simulink model "ModID_R2018a"  (R2018a)
settings: Solver=VariableStepAuto  StartTime=0.0  StopTime=10.0  RelTol=1e-3
values from neighbouring files (symbols this model uses):
  matrcomp =     [theta_sim_nonlinv2.mat]
libraries: dspinverses x1
settings Model: Creator=jannekeblok  LastModifiedBy=jessi
settings DebuggingCC: LibraryContextMissingDiagnostic=warning
settings CodeAppCC: StateflowObjectComments=on

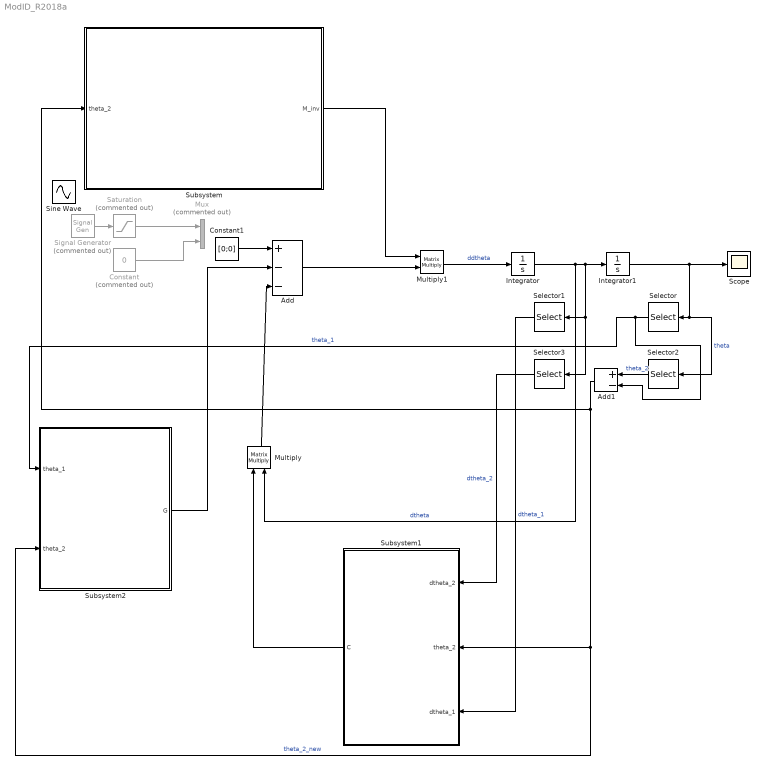
== system ModID_R2018a ==
  Add : Sum  Inputs=+--
  Add1 : Sum  Inputs=+-
  Constant : Constant  Commented=on  Value=0
  Constant1 : Constant  Value=[0;0]
  Integrator : Integrator
  Integrator1 : Integrator  InitialCondition=[pi;3/2*pi]
  Multiply : Product  Multiplication=Matrix(*)
  Multiply1 : Product  Multiplication=Matrix(*)
  Mux : Mux  Commented=on  Inputs=2
  Saturation : Saturate  Commented=on  UpperLimit=1  LowerLimit=-1
  Scope : Scope
  Selector : Selector  InputPortWidth=2  IndexOptions=Index vector (dialog)  Indices=[1]  OutputSizes=1
  Selector1 : Selector  InputPortWidth=2  IndexOptions=Index vector (dialog)  Indices=[1]  OutputSizes=1
  Selector2 : Selector  InputPortWidth=2  IndexOptions=Index vector (dialog)  Indices=[2]  OutputSizes=1
  Selector3 : Selector  InputPortWidth=2  IndexOptions=Index vector (dialog)  Indices=[2]  OutputSizes=1
  Signal Generator : SignalGenerator  Commented=on  Amplitude=0.3*1  Units=rad/sec
  Sine Wave : Sin  SampleTime=0
  Subsystem : Subsystem
  Subsystem1 : Subsystem
  Subsystem2 : Subsystem
  wires:
  Multiply/1 -> Add/3
  Subsystem/1(M_inv) -> Multiply1/1
  Add/1 -> Multiply1/2
  Subsystem1/1(C) -> Multiply/1
  Integrator/1 -> Multiply/2, Selector1/1, Selector3/1, Integrator1/1  "dtheta"
  Selector/1 -> Add1/2, Subsystem2/1(theta_1)  "theta_1"
  Multiply1/1 -> Integrator/1  "ddtheta"
  Constant/1 -> Mux/2
  Selector1/1 -> Subsystem1/3(dtheta_1)  "dtheta_1"
  Constant1/1 -> Add/1
  Selector2/1 -> Add1/1  "theta_2"
  Selector3/1 -> Subsystem1/1(dtheta_2)  "dtheta_2"
  Signal Generator/1 -> Saturation/1
  Integrator1/1 -> Scope/1, Selector2/1, Selector/1  "theta"
  Subsystem2/1(G) -> Add/2
  Saturation/1 -> Mux/1
  Add1/1 -> Subsystem2/2("theta_2 "), Subsystem1/2(theta_2), Subsystem/1("theta_2 ")  "theta_2_new"

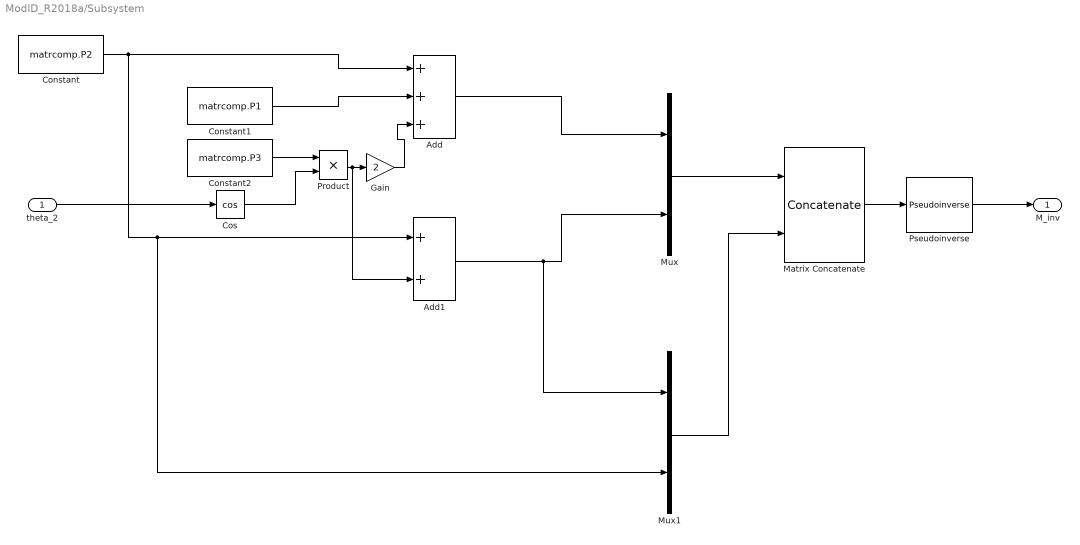
== system ModID_R2018a/Subsystem ==
  "theta_2 " : Inport
  Add : Sum  Inputs=+++
  Add1 : Sum
  Constant : Constant  Value=matrcomp.P2
  Constant1 : Constant  Value=matrcomp.P1
  Constant2 : Constant  Value=matrcomp.P3
  Cos : Trigonometry  Operator=cos
  Gain : Gain  Gain=2
  Matrix Concatenate : Concatenate  Mode=Multidimensional array  ConcatenateDimension=2
  Mux : Mux  Inputs=2
  Mux1 : Mux  Inputs=2
  Product : Product
  Pseudoinverse : dspinverses/Pseudoinverse  wanterr=off  SimulateUsing=Interpreted execution
      settings: SourceProductName=DSP System Toolbox  SourceProductBaseCode=DS
  M_inv : Outport
  wires:
  Matrix Concatenate/1 -> Pseudoinverse/1
  Product/1 -> Add1/2, Gain/1
  Mux/1 -> Matrix Concatenate/1
  Cos/1 -> Product/2
  "theta_2 "/1 -> Cos/1
  Gain/1 -> Add/3
  Add/1 -> Mux/1
  Pseudoinverse/1 -> M_inv/1
  Constant1/1 -> Add/2
  Constant2/1 -> Product/1
  Add1/1 -> Mux1/1, Mux/2
  Constant/1 -> Mux1/2, Add1/1, Add/1
  Mux1/1 -> Matrix Concatenate/2

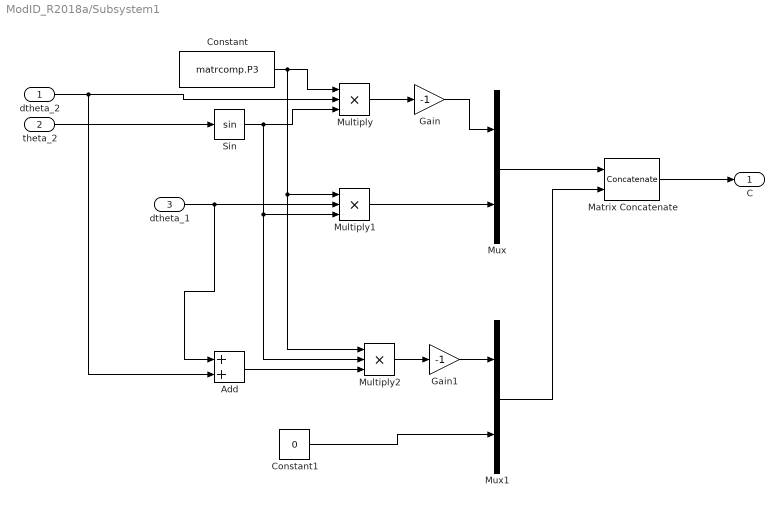
== system ModID_R2018a/Subsystem1 ==
  dtheta_2 : Inport
  theta_2 : Inport  Port=2
  dtheta_1 : Inport  Port=3
  Add : Sum
  Constant : Constant  Value=matrcomp.P3
  Constant1 : Constant  Value=0
  Gain : Gain  Gain=-1
  Gain1 : Gain  Gain=-1
  Matrix Concatenate : Concatenate  Mode=Multidimensional array  ConcatenateDimension=2
  Multiply : Product  Inputs=3
  Multiply1 : Product  Inputs=3
  Multiply2 : Product  Inputs=3
  Mux : Mux  Inputs=2
  Mux1 : Mux  Inputs=2
  Sin : Trigonometry
  C : Outport
  wires:
  Gain1/1 -> Mux1/1
  Mux1/1 -> Matrix Concatenate/2
  Add/1 -> Multiply2/3
  Multiply2/1 -> Gain1/1
  dtheta_1/1 -> Add/1, Multiply1/2
  Multiply/1 -> Gain/1
  Gain/1 -> Mux/1
  Matrix Concatenate/1 -> C/1
  Multiply1/1 -> Mux/2
  Constant/1 -> Multiply1/1, Multiply2/1, Multiply/1
  Mux/1 -> Matrix Concatenate/1
  Constant1/1 -> Mux1/2
  dtheta_2/1 -> Add/2, Multiply/2
  theta_2/1 -> Sin/1
  Sin/1 -> Multiply1/3, Multiply2/2, Multiply/3

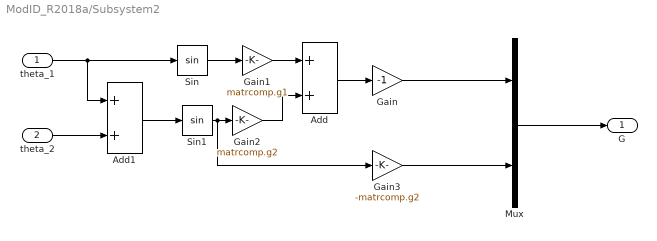
== system ModID_R2018a/Subsystem2 ==
  theta_1 : Inport
  "theta_2 " : Inport  Port=2
  Add : Sum
  Add1 : Sum
  Gain : Gain  Gain=-1
  Gain1 : Gain  Gain=matrcomp.g1
  Gain2 : Gain  Gain=matrcomp.g2
  Gain3 : Gain  Gain=-matrcomp.g2
  Mux : Mux  Inputs=2
  Sin : Trigonometry
  Sin1 : Trigonometry
  G : Outport
  wires:
  Gain2/1 -> Add/2
  Mux/1 -> G/1
  Add1/1 -> Sin1/1
  Gain3/1 -> Mux/2
  Add/1 -> Gain/1
  Sin/1 -> Gain1/1
  Sin1/1 -> Gain3/1, Gain2/1
  Gain1/1 -> Add/1
  Gain/1 -> Mux/1
  "theta_2 "/1 -> Add1/2
  theta_1/1 -> Sin/1, Add1/1
